simulink model "AMR_rcuControlUnit_24a"  (R2024a)
settings: configuration reference "SharedConfig" (kept outside this file)
undefined symbols (not defined in the file): max_RCU_speed
libraries: simulink x5
settings Model: DataDictionary=configuration_dictionary.sldd  Creator=matlab.cut  LastModifiedBy=matlab.cut
settings ConfigSetRef: SourceName=SharedConfig

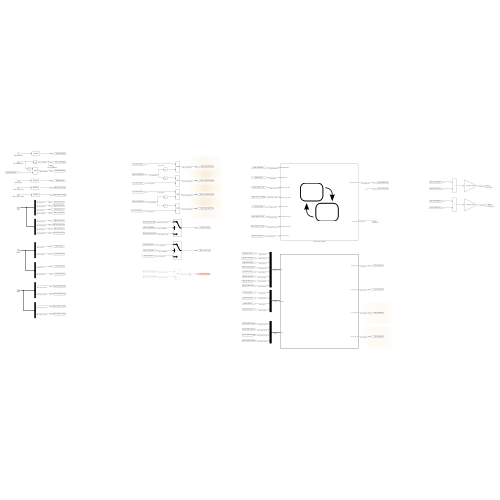
[thumbnail: Simulink's stored preview of the top-level diagram]
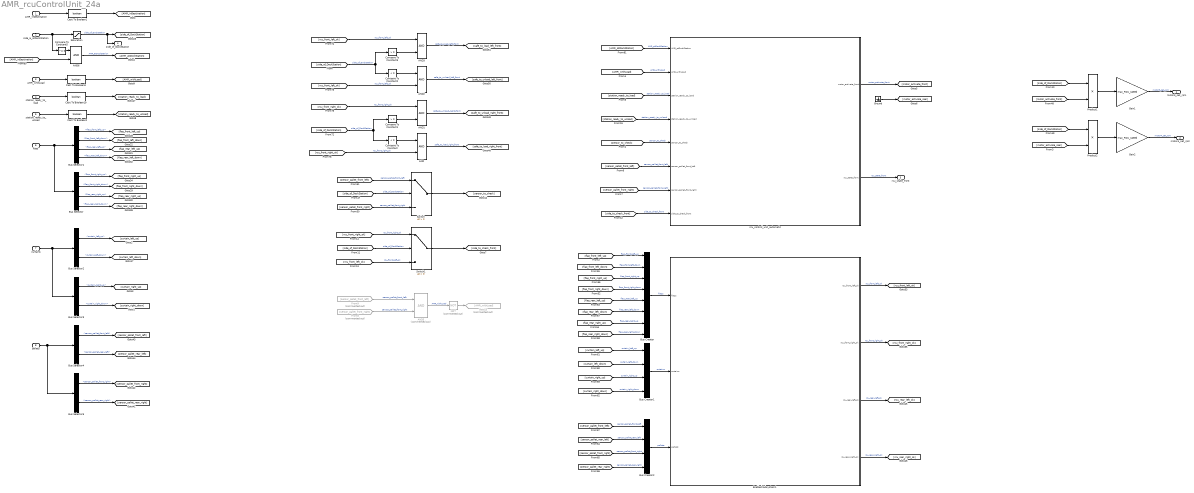
== system AMR_rcuControlUnit_24a ==
  AMR_inDestination : Inport
  side_&_atDockStation : Inport  Port=2
  AMR_whitLoad : Inport  Port=3
  station_ready_to_load : Inport  Port=4
  station_ready_to_unload : Inport  Port=5
  flaps : Inport  Port=6  OutDataTypeStr=Bus: IOs_flaps_bool
  curtains : Inport  Port=7  OutDataTypeStr=Bus: IOs_curtains_bool
  pallets : Inport  Port=8  OutDataTypeStr=Bus: IOs_pallets_bool
  AND{,1..3,6} (5 alike) : Logic  AllPortsSameDT=off  OutDataTypeStr=boolean
  AND5 : Logic  Commented=on  AllPortsSameDT=off  OutDataTypeStr=boolean
  Bus Creator : BusCreator  Inputs=8
  Bus Creator1 : BusCreator  Inputs=4
  Bus Creator2 : BusCreator  Inputs=4
  Bus Selector : BusSelector  OutputSignals=flap_front_right_up,flap_front_right_down,flap_rear_right_up,flap_rear_right_down
  Bus Selector1 : BusSelector  OutputSignals=flap_front_left_up,flap_front_left_down,flap_rear_left_up,flap_rear_left_down
  Bus Selector2 : BusSelector  OutputSignals=curtain_left_up,curtain_left_down
  Bus Selector3 : BusSelector  OutputSignals=curtain_right_up,curtain_right_down
  Bus Selector4 : BusSelector  OutputSignals=sensor_pallet_front_left,sensor_pallet_rear_left
  Bus Selector5 : BusSelector  OutputSignals=sensor_pallet_front_right,sensor_pallet_rear_right
  Cast To Boolean{1..3,19} (4 alike) : DataTypeConversion  OutDataTypeStr=boolean  SaturateOnIntegerOverflow=off  RndMeth=Floor
  Compare To Constant : simulink/Logic and Bit Operations/Compare To Constant  relop=<  const=0  OutDataTypeStr=boolean
  Compare To Constant1 : simulink/Logic and Bit Operations/Compare To Constant  relop=>  const=0  OutDataTypeStr=boolean
  Compare To Constant2 : simulink/Logic and Bit Operations/Compare To Constant  relop=<  const=0  OutDataTypeStr=boolean
  Compare To Constant3 : simulink/Logic and Bit Operations/Compare To Constant  relop=>  const=0  OutDataTypeStr=boolean
  Compare To Constant5 : simulink/Logic and Bit Operations/Compare To Constant  relop=~=  const=0  OutDataTypeStr=boolean
  Enabled Subsystem1 : Subsystem  TreatAsAtomicUnit=on
  From8 : From  Commented=on  GotoTag=sensor_pallet_front_right
  From9 : From  Commented=on  GotoTag=sensor_pallet_front_left
  Gain1 : Gain  Gain=max_RCU_speed
  Gain2 : Gain  Gain=max_RCU_speed
  Goto25 : Goto  Commented=on  GotoTag=AMR_withLoad
  Ground : Ground
  NOT : Logic  Commented=on  Operator=NOT  IconShape=distinctive  AllPortsSameDT=off  OutDataTypeStr=boolean
  Product1 : Product
  Product2 : Product
  Saturation : Saturate  UpperLimit=1  LowerLimit=-1
  Switch : Switch  Criteria=u2 > Threshold  SaturateOnIntegerOverflow=off  InputSameDT=off
  Switch1 : Switch  Criteria=u2 > Threshold  SaturateOnIntegerOverflow=off  InputSameDT=off
  rcu_control_unit_automatic : Stateflow chart  TreatAsAtomicUnit=on
      settings: PortSchema="{\"entries\":[{\"content\":{\"sides\":[{\"content\":{\"connectorIds\":[\"In1\",\"In2\",\"In7\",\"In8\",\"In6\",\"In3\",\"In4\",\"In5\"]},\"type\":\"ConnectorPlacement.EquallySpacedRectSide\",\"uuid\":\"58ff1d1e-d919-48b2-9a3c-17793bae4070\"},{\"content\":{\"connectorIds\":[\"Out1\",\"Out2\"],\"side\":\"RIGHT\"},\"type\":\"ConnectorPlacement.EquallySpacedRectSide\",\"uuid\":\"96e6ef9e-cd68-4a53-95c8-269ebe0f7ef0\"},{\"content\":{\"side\":\"TOP\"},\"type\":\"ConnectorPlacement.EquallySpacedRectSide\",\"uuid\":\"483355b4-8761-4fc4-a009-24c3824dab6c\"}]},\"type\":\"ConnectorPlacement.EquallySpacedConnector\",\"uuid\":\"a15f46ca-3a58-4377-bdb0-a873cbd87e71\"}],\"packageUris\":[\"http://schema.mathworks.com/mf0/Connector/R2020b\"],\"version\":\"1.0\"}"
  motor3_set_rpm : Outport
  motor4_set_rpm : Outport  Port=2
  rcu_state_front : Outport  Port=3
  side_of_DockStation : Outport  Port=4
  wires:
  Enabled Subsystem1/4(rcu_rear_right_ok) -> [rcu_rear_right_ok]  "rcu_rear_right_ok"
  Enabled Subsystem1/2(rcu_front_right_ok) -> [rcu_front_right_ok]  "rcu_front_right_ok"
  Enabled Subsystem1/1(rcu_front_left_ok) -> [rcu_front_left_ok]  "rcu_front_left_ok"
  Enabled Subsystem1/3(rcu_rear_left_ok) -> [rcu_rear_left_ok]  "rcu_rear_left_ok"
  [sensor_to_check] -> rcu_control_unit_automatic/6(sensor_to_check)  "sensor_to_check"
  [AMR_withLoad] -> rcu_control_unit_automatic/2(AMR_withLoad)  "AMR_withLoad"
  [AMR_atDockStation] -> rcu_control_unit_automatic/1(AMR_atDockStation)  "AMR_atDockStation"
  [sensor_pallet_front_left] -> rcu_control_unit_automatic/3(sensor_pallet_front_left)  "sensor_pallet_front_left"
  [sensor_pallet_front_right] -> rcu_control_unit_automatic/4(sensor_pallet_front_right)  "sensor_pallet_front_right"
  [side_to_check_front] -> rcu_control_unit_automatic/5(side_to_check_front)  "side_to_check_front"
  [rcu_front_left_ok] -> AND3/1  "rcu_front_left_ok"
  [rcu_front_right_ok] -> AND/2  "rcu_front_right_ok"
  Compare To Constant/1 -> AND/1
  AND1/1 -> [safe_to_unload_right_front]  "safe_to_unload_right_front"
  [side_of_DockStation] -> Compare To Constant3/1, Compare To Constant2/1  "side_of_DockStation"
  Compare To Constant2/1 -> AND2/1
  AND2/1 -> [safe_to_unload_left_front]  "safe_to_unload_left_front"
  [sensor_pallet_front_left] -> Switch/1  "sensor_pallet_front_left"
  AND3/1 -> [safe_to_load_left_front]  "safe_to_load_left_front"
  [sensor_pallet_front_right] -> Switch/3  "sensor_pallet_front_right"
  Compare To Constant1/1 -> AND1/2
  Switch/1 -> [sensor_to_check]
  [side_of_DockStation] -> Switch/2  "side_of_DockStation"
  [side_of_DockStation] -> Compare To Constant/1, Compare To Constant1/1  "side_of_DockStation"
  [rcu_front_right_ok] -> AND1/1  "rcu_front_right_ok"
  From9/1 -> AND5/1  "sensor_pallet_front_left"
  [rcu_front_left_ok] -> AND2/2  "rcu_front_left_ok"
  Compare To Constant3/1 -> AND3/2
  AND/1 -> [safe_to_load_right_front]  "safe_to_load_right_front"
  AND5/1 -> NOT/1  "AMR_withLoad"
  Bus Selector4/2 -> [sensor_pallet_rear_left]  "<sensor_pallet_rear_left>"
  Bus Selector5/2 -> [sensor_pallet_rear_right]  "<sensor_pallet_rear_right>"
  Bus Selector4/1 -> [sensor_pallet_front_left]  "<sensor_pallet_front_left>"
  Bus Selector5/1 -> [sensor_pallet_front_right]  "<sensor_pallet_front_right>"
  pallets/1 -> Bus Selector5/1, Bus Selector4/1
  Bus Selector3/1 -> [curtain_right_up]  "<curtain_right_up>"
  Bus Selector1/4 -> [flap_rear_left_down]  "<flap_rear_left_down>"
  Bus Selector2/1 -> [curtain_left_up]  "<curtain_left_up>"
  Bus Selector/3 -> [flap_rear_right_up]  "<flap_rear_right_up>"
  Bus Selector1/2 -> [flap_front_left_down]  "<flap_front_left_down>"
  Bus Selector/4 -> [flap_rear_right_down]  "<flap_rear_right_down>"
  Bus Selector3/2 -> [curtain_right_down]  "<curtain_right_down>"
  flaps/1 -> Bus Selector/1, Bus Selector1/1
  Bus Selector2/2 -> [curtain_left_down]  "<curtain_left_down>"
  Bus Selector1/3 -> [flap_rear_left_up]  "<flap_rear_left_up>"
  Bus Selector1/1 -> [flap_front_left_up]  "<flap_front_left_up>"
  Bus Selector/1 -> [flap_front_right_up]  "<flap_front_right_up>"
  curtains/1 -> Bus Selector3/1, Bus Selector2/1
  Bus Selector/2 -> [flap_front_right_down]  "<flap_front_right_down>"
  Saturation/1 -> side_of_DockStation/1, [side_of_DockStation]  "side_of_DockStation"
  [AMR_inDestination] -> AND6/2
  Compare To Constant5/1 -> AND6/1
  AND6/1 -> [AMR_atDockStation]  "AMR_atDockStation"
  side_&_atDockStation/1 -> Compare To Constant5/1, Saturation/1
  Cast To Boolean19/1 -> [station_ready_to_load]
  station_ready_to_load/1 -> Cast To Boolean19/1
  rcu_control_unit_automatic/1(motor_activate_front) -> [motor_activate_front]  "motor_activate_front"
  rcu_control_unit_automatic/2(rcu_state_front) -> rcu_state_front/1  "rcu_state_front"
  Ground/1 -> [motor_activate_rear]
  AMR_inDestination/1 -> Cast To Boolean1/1
  Cast To Boolean1/1 -> [AMR_inDestination]
  [curtain_left_up] -> Bus Creator1/1  "curtain_left_up"
  Bus Creator2/1 -> Enabled Subsystem1/3(pallets)  "pallets"
  [flap_rear_left_up] -> Bus Creator/5  "flap_rear_left_up"
  [flap_rear_left_down] -> Bus Creator/6  "flap_rear_left_down"
  [sensor_pallet_front_left] -> Bus Creator2/1  "sensor_pallet_front_left"
  [curtain_right_up] -> Bus Creator1/3  "curtain_right_up"
  [sensor_pallet_rear_left] -> Bus Creator2/2  "sensor_pallet_rear_left"
  Bus Creator1/1 -> Enabled Subsystem1/2(curtains)  "curtains"
  [sensor_pallet_front_right] -> Bus Creator2/3  "sensor_pallet_front_right"
  [curtain_left_down] -> Bus Creator1/2  "curtain_left_down"
  Bus Creator/1 -> Enabled Subsystem1/1(flaps)  "flaps"
  [flap_front_right_up] -> Bus Creator/3  "flap_front_right_up"
  [flap_front_left_up] -> Bus Creator/1  "flap_front_left_up"
  [flap_rear_right_up] -> Bus Creator/7  "flap_rear_right_up"
  [curtain_right_down] -> Bus Creator1/4  "curtain_right_down"
  [flap_front_left_down] -> Bus Creator/2  "flap_front_left_down"
  [flap_front_right_down] -> Bus Creator/4  "flap_front_right_down"
  [flap_rear_right_down] -> Bus Creator/8  "flap_rear_right_down"
  [sensor_pallet_rear_right] -> Bus Creator2/4  "sensor_pallet_rear_right"
  Product1/1 -> Gain1/1
  [side_of_DockStation] -> Product1/1
  Gain2/1 -> motor4_set_rpm/1  "motor4_set_rpm"
  Gain1/1 -> motor3_set_rpm/1  "motor3_set_rpm"
  [side_of_DockStation] -> Product2/1
  Product2/1 -> Gain2/1
  [motor_activate_front] -> Product1/2
  [motor_activate_rear] -> Product2/2
  [side_of_DockStation] -> Switch1/2  "side_of_DockStation"
  Switch1/1 -> [side_to_check_front]
  [rcu_front_left_ok] -> Switch1/3  "rcu_front_left_ok"
  [rcu_front_right_ok] -> Switch1/1  "rcu_front_right_ok"
  From8/1 -> AND5/2  "sensor_pallet_front_right"
  [station_ready_to_load] -> rcu_control_unit_automatic/7(station_ready_to_load)  "station_ready_to_load"
  station_ready_to_unload/1 -> Cast To Boolean2/1
  [station_ready_to_unload] -> rcu_control_unit_automatic/8(station_ready_to_unload)  "station_ready_to_unload"
  NOT/1 -> Goto25/1
  Cast To Boolean2/1 -> [station_ready_to_unload]
  AMR_whitLoad/1 -> Cast To Boolean3/1
  Cast To Boolean3/1 -> [AMR_withLoad]

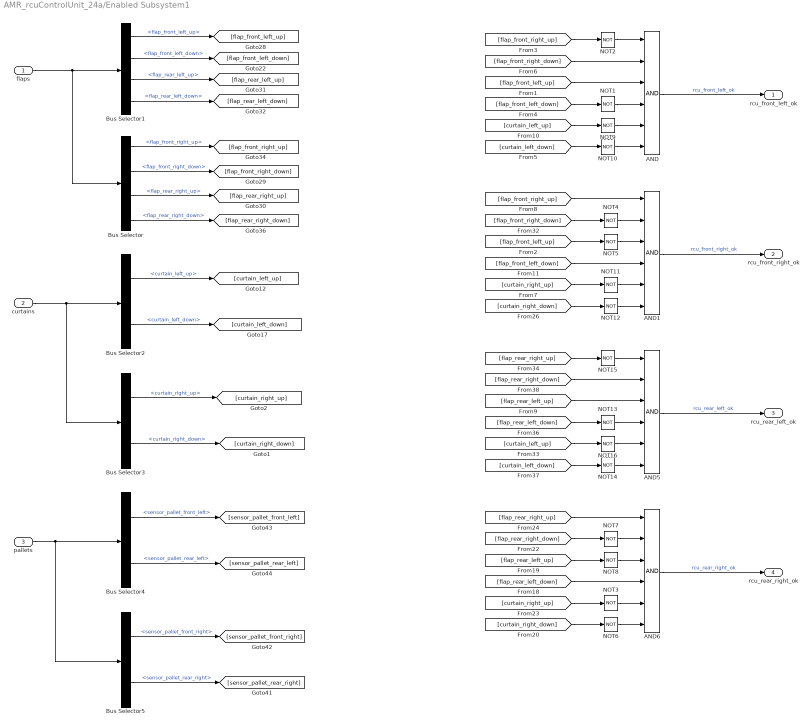
== system AMR_rcuControlUnit_24a/Enabled Subsystem1 ==
  flaps : Inport
  curtains : Inport  Port=2
  pallets : Inport  Port=3
  AND{,1,5..6} (4 alike) : Logic  Inputs=6  AllPortsSameDT=off  OutDataTypeStr=boolean
  Bus Selector : BusSelector  OutputSignals=flap_front_right_up,flap_front_right_down,flap_rear_right_up,flap_rear_right_down
  Bus Selector1 : BusSelector  OutputSignals=flap_front_left_up,flap_front_left_down,flap_rear_left_up,flap_rear_left_down
  Bus Selector2 : BusSelector  OutputSignals=curtain_left_up,curtain_left_down
  Bus Selector3 : BusSelector  OutputSignals=curtain_right_up,curtain_right_down
  Bus Selector4 : BusSelector  OutputSignals=sensor_pallet_front_left,sensor_pallet_rear_left
  Bus Selector5 : BusSelector  OutputSignals=sensor_pallet_front_right,sensor_pallet_rear_right
  NOT{1..16} (16 alike) : Logic  Operator=NOT  IconShape=distinctive  AllPortsSameDT=off  OutDataTypeStr=boolean
  rcu_front_left_ok : Outport
  rcu_front_right_ok : Outport  Port=2
  rcu_rear_left_ok : Outport  Port=3
  rcu_rear_right_ok : Outport  Port=4
  wires:
  [curtain_left_down] -> NOT10/1
  [curtain_left_up] -> NOT9/1
  NOT4/1 -> AND1/2
  NOT5/1 -> AND1/3
  [flap_front_right_up] -> AND1/1
  [flap_front_left_up] -> NOT5/1
  [flap_front_left_down] -> AND1/4
  [flap_front_right_down] -> NOT4/1
  [flap_front_right_up] -> NOT2/1
  [flap_front_right_down] -> AND/2
  [flap_front_left_down] -> NOT1/1
  NOT1/1 -> AND/4
  [flap_front_left_up] -> AND/3
  NOT2/1 -> AND/1
  flaps/1 -> Bus Selector/1, Bus Selector1/1
  Bus Selector1/1 -> [flap_front_left_up]  "<flap_front_left_up>"
  Bus Selector1/2 -> [flap_front_left_down]  "<flap_front_left_down>"
  Bus Selector1/3 -> [flap_rear_left_up]  "<flap_rear_left_up>"
  Bus Selector1/4 -> [flap_rear_left_down]  "<flap_rear_left_down>"
  Bus Selector/1 -> [flap_front_right_up]  "<flap_front_right_up>"
  Bus Selector/2 -> [flap_front_right_down]  "<flap_front_right_down>"
  Bus Selector/3 -> [flap_rear_right_up]  "<flap_rear_right_up>"
  Bus Selector/4 -> [flap_rear_right_down]  "<flap_rear_right_down>"
  curtains/1 -> Bus Selector3/1, Bus Selector2/1
  Bus Selector2/2 -> [curtain_left_down]  "<curtain_left_down>"
  Bus Selector2/1 -> [curtain_left_up]  "<curtain_left_up>"
  Bus Selector3/1 -> [curtain_right_up]  "<curtain_right_up>"
  Bus Selector3/2 -> [curtain_right_down]  "<curtain_right_down>"
  pallets/1 -> Bus Selector5/1, Bus Selector4/1
  Bus Selector4/1 -> [sensor_pallet_front_left]  "<sensor_pallet_front_left>"
  Bus Selector4/2 -> [sensor_pallet_rear_left]  "<sensor_pallet_rear_left>"
  Bus Selector5/1 -> [sensor_pallet_front_right]  "<sensor_pallet_front_right>"
  Bus Selector5/2 -> [sensor_pallet_rear_right]  "<sensor_pallet_rear_right>"
  AND/1 -> rcu_front_left_ok/1  "rcu_front_left_ok"
  NOT9/1 -> AND/5
  NOT10/1 -> AND/6
  NOT11/1 -> AND1/5
  NOT12/1 -> AND1/6
  [curtain_right_up] -> NOT11/1
  [curtain_right_down] -> NOT12/1
  [flap_rear_left_down] -> NOT13/1
  [flap_rear_right_up] -> NOT15/1
  [curtain_left_up] -> NOT16/1
  [curtain_left_down] -> NOT14/1
  NOT15/1 -> AND5/1
  NOT13/1 -> AND5/4
  NOT16/1 -> AND5/5
  NOT14/1 -> AND5/6
  [flap_rear_right_down] -> AND5/2
  [flap_rear_left_up] -> AND5/3
  AND5/1 -> rcu_rear_left_ok/1  "rcu_rear_left_ok"
  AND1/1 -> rcu_front_right_ok/1  "rcu_front_right_ok"
  [curtain_right_down] -> NOT6/1
  [curtain_right_up] -> NOT3/1
  NOT6/1 -> AND6/6
  NOT3/1 -> AND6/5
  [flap_rear_right_down] -> NOT7/1
  [flap_rear_left_down] -> AND6/4
  [flap_rear_left_up] -> NOT8/1
  [flap_rear_right_up] -> AND6/1
  NOT8/1 -> AND6/3
  NOT7/1 -> AND6/2
  AND6/1 -> rcu_rear_right_ok/1  "rcu_rear_right_ok"

== stateflow chart AMR_rcuControlUnit_24a/rcu_control_unit_automatic ==
  state RCU_idle
    entry:
    rcu_state_front = 0;
  state pre_loading
    entry:
    rcu_state_front = 1;
  state pre_unloading
    entry:
    rcu_state_front = -1;
  state loading
    entry:
    rcu_state_front = 2;
    motor_activate_front=1;
    exit:
    motor_activate_front=0;
  state unloading
    entry:
    rcu_state_front = -2;
    motor_activate_front=-1;
    exit:
    motor_activate_front = 0;
  (default) -> RCU_idle
  (junction 111) -> RCU_idle
  (junction 110) -> (junction 111)
  RCU_idle -> (junction 224) : [AMR_atDockStation==TRUE]
  (junction 224) -> (junction 225) [order 2] : [AMR_withLoad==FALSE &&...
      | station_ready_to_load==TRUE]
  (junction 224) -> (junction 226) [order 1] : [AMR_withLoad==TRUE &&...
      | station_ready_to_unload==TRUE]
  (junction 225) -> pre_loading
  (junction 226) -> pre_unloading
  pre_loading -> (junction 221) [order 2] : [AMR_withLoad==TRUE]
  (junction 221) -> (junction 172)
  pre_unloading -> (junction 206) [order 2] : [AMR_withLoad==FALSE]
  (junction 206) -> (junction 209)
  pre_loading -> loading [order 1] : [side_to_check_front == 1 &&...
      | station_ready_to_load==TRUE]
  pre_unloading -> unloading [order 1] : [side_to_check_front == 1 &&...
      | station_ready_to_unload==TRUE]
  loading -> (junction 108) : [(sensor_to_check==TRUE &&...
      | AMR_withLoad==TRUE) ||...
      | side_to_check_front==0]
  unloading -> (junction 109) : [(station_ready_to_unload==FALSE && ...
      | sensor_pallet_front_left == 1 && ...
      | sensor_pallet_front_right == 1) || ...
      | side_to_check_front == 0 ]
  (junction 209) -> (junction 109)
  (junction 109) -> (junction 172)
  (junction 108) -> (junction 110)
  (junction 172) -> (junction 108)
  data: AMR_atDockStation input; TRUE constant double =1; FALSE constant double =0; AMR_withLoad input =0; motor_activate_front output; rcu_state_front output size=1 =0; sensor_pallet_front_left input; sensor_pallet_front_right input; side_to_check_front input; sensor_to_check input; station_ready_to_load input; station_ready_to_unload input
